simulink model "compass"  (R2021a)
settings: Solver=VariableStepAuto  StartTime=0.0  StopTime=100  RelTol=1e-4
values from neighbouring files (symbols this model uses):
  a = 1    [Main.m]
  b = 2*eta/w    (= 0.0512623349994)    [Main.m]
  c = 1/w^2    (= 0.153787004998)    [Main.m]
  d = k    (= 2)    [Main.m]
undefined symbols (not defined in the file or in its folder): heading
settings Model: Creator=zd012  LastModifiedBy=zd012

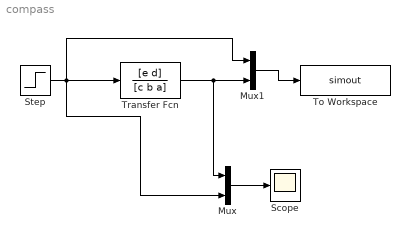
== system compass ==
  Mux : Mux  Inputs=2
  Mux1 : Mux  Inputs=2
  Scope : Scope
  Step : Step  After=heading  SampleTime=0
  To Workspace : ToWorkspace  VariableName=simout  SaveFormat=Timeseries  SampleTime=-1
  Transfer Fcn : TransferFcn  Numerator=[e d]  Denominator=[c b a]
  wires:
  Step/1 -> Mux1/1, Mux/2, Transfer Fcn/1
  Transfer Fcn/1 -> Mux1/2, Mux/1
  Mux/1 -> Scope/1
  Mux1/1 -> To Workspace/1
